simulink model "DC_Motor_model_closed_loop"  (R2026a)
settings: Solver=VariableStepAuto
model workspace (MAT data in the model file):
  B = Simulink.Parameter
  B.Value = 0.0001
  B.Complexity = 'real'
  B.Dimensions = [1 1]
  B.DataType = 'auto'
  J = Simulink.Parameter
  J.Value = 5e-05
  J.Complexity = 'real'
  J.Dimensions = [1 1]
  J.DataType = 'auto'
  Ke = Simulink.Parameter
  Ke.Value = 0.012
  Ke.Complexity = 'real'
  Ke.Dimensions = [1 1]
  Ke.DataType = 'auto'
  Kt = Simulink.Parameter
  Kt.Value = 0.012
  Kt.Complexity = 'real'
  Kt.Dimensions = [1 1]
  Kt.DataType = 'auto'
  L = Simulink.Parameter
  L.Value = 0.01
  L.Complexity = 'real'
  L.Dimensions = [1 1]
  L.DataType = 'auto'
  R = Simulink.Parameter
  R.Value = 5
  R.Complexity = 'real'
  R.Dimensions = [1 1]
  R.DataType = 'auto'
  TL = Simulink.Parameter
  TL.Value = 0
  TL.Complexity = 'real'
  TL.Dimensions = [1 1]
  TL.DataType = 'auto'
libraries: slpidlib x1

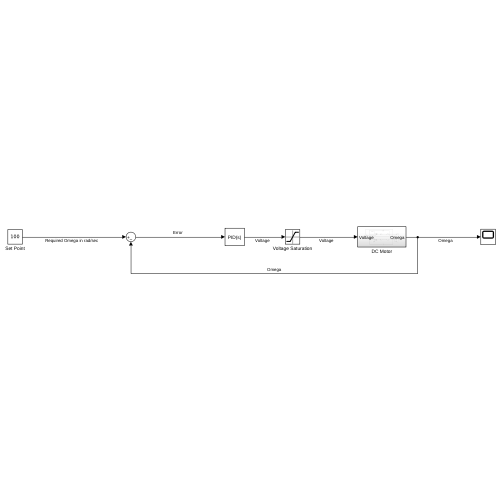
[thumbnail: Simulink's stored preview of the top-level diagram]
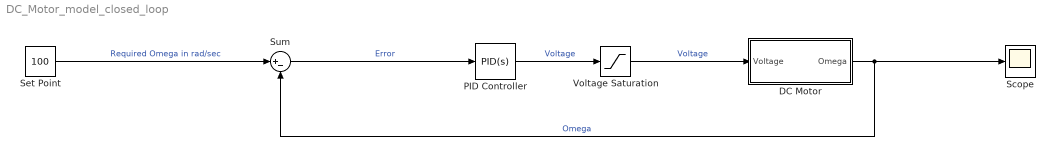
== system DC_Motor_model_closed_loop ==
  DC Motor : Subsystem
  PID Controller : slpidlib/PID Controller  Controller=PID  Form=Parallel  TimeDomain=Continuous-time  UseExternalTs=off  SampleTime=-1  IntegratorMethod=Forward Euler  FilterMethod=Forward Euler  ControllerParametersSource=internal  P=0.04  I=0.2  UseKiTs=off  D=0  UseExternalDerivativeSource=off  N=100  UseFilter=on  TunerSelectOption=Transfer Function Based (PID Tuner App)  InitialConditionSource=internal  InitialConditionForIntegrator=0  InitialConditionForFilter=0  DifferentiatorICPrevScaledInput=0  ExternalReset=none  TrackingMode=off  Kt=1  LimitOutput=off  SatLimitsSource=internal  UpperSaturationLimit=inf  LowerSaturationLimit=-inf  LinearizeAsGain=on  AntiWindupMode=none  Kb=1  LimitIntegrator=off  UpperIntegratorSaturationLimit=inf  LowerIntegratorSaturationLimit=-inf  POutMin=[]  POutMax=[]  IOutMin=[]  IOutMax=[]  DOutMin=[]  DOutMax=[]  NOutMin=[]  NOutMax=[]  SumOutMin=[]  SumOutMax=[]  SaturationOutMin=[]  SaturationOutMax=[]  PParamMin=[]  PParamMax=[]  IParamMin=[]  IParamMax=[]  DParamMin=[]  DParamMax=[]  NParamMin=[]  NParamMax=[]  KbParamMin=[]  KbParamMax=[]  KtParamMin=[]  KtParamMax=[]  KbOutMin=[]  KbOutMax=[]  KtOutMin=[]  KtOutMax=[]  IntegratorOutMin=[]  IntegratorOutMax=[]  FilterOutMin=[]  FilterOutMax=[]  SumI1OutMin=[]  SumI1OutMax=[]  SumI2OutMin=[]  SumI2OutMax=[]  SumI3OutMin=[]  SumI3OutMax=[]  SumI4OutMin=[]  SumI4OutMax=[]  SumDOutMin=[]  SumDOutMax=[]  DifferentiatorOutMin=[]  DifferentiatorOutMax=[]  FilterDiffOutCoefMin=[]  FilterDiffOutCoefMax=[]  ReciprocalOutMin=[]  ReciprocalOutMax=[]  SumDenOutMin=[]  SumDenOutMax=[]  SumNumOutMin=[]  SumNumOutMax=[]  DivideOutMin=[]  DivideOutMax=[]  UdiffTsProdOutMin=[]  UdiffTsProdOutMax=[]  NTsProdOutMin=[]  NTsProdOutMax=[]  UintegralTsProdOutMin=[]  UintegralTsProdOutMax=[]  UngainTsProdOutMin=[]  UngainTsProdOutMax=[]  ClampingZeroOutDataTypeStr=Inherit: Inherit via back propagation  ClampingZeroOutMin=[]  ClampingZeroOutMax=[]  FilterDenConstantOutDataTypeStr=Inherit: Inherit via back propagation  FilterDenConstantOutMin=[]  FilterDenConstantOutMax=[]  PCopyOutDataTypeStr=Inherit: Inherit via back propagation  PCopyOutMin=[]  PCopyOutMax=[]  NCopyOutDataTypeStr=Inherit: Inherit via back propagation  NCopyOutMin=[]  NCopyOutMax=[]  IntegratorContinuousStateAttributes=''  IntegratorStateMustResolveToSignalObject=off  IntegratorRTWStateStorageClass=Auto  FilterContinuousStateAttributes=''  FilterStateMustResolveToSignalObject=off  FilterRTWStateStorageClass=Auto  ParallelPVariant=InternalParameters  IdealPVariant=Disabled  IVariant=InternalParameters  DVariant=InternalParameters  IntegratorVariant=Continuous  SatVariant=Disabled  AWVariant=Passthrough  PCopyVariant=Disabled  TRVariant=Disabled  FdbkBlocksVariant=Forward  IdealPFdbkVariant=Disabled  SatFdbkVariant=Disabled  DerivativeFilterVariant=ContFilter  NVariant=InternalParameters  NCopyVariant=Disabled  FilterICVariant=InternalICsFilter  IntegratorICVariant=InternalICs  ExternalResetVariant=Disabled  TRSumVariant=Passthrough  SumFdbkVariant=Disabled  SumVariant=Sum_PID  TsampFilterVariant=InternalTs  TsampNgainVariant=Passthrough  TsampIntegralVariant=Disabled_SignalSpec  ExternalSaturationOutDataTypeStr=Inherit: Same as second input  DerivativeSourceVariant=ErrorSignal  PreIntVariant=InternalPreInt
  Scope : Scope
      settings: ActiveDisplayYMinimum=-13.144303855447449  ActiveDisplayYMaximum=118.29873469902707  DataLoggingVariableName=ScopeData2
  Set Point : Constant  Value=100
  Sum : Sum  Inputs=|+-
  Voltage Saturation : Saturate  UpperLimit=12  LowerLimit=0
  wires:
  Sum/1 -> PID Controller/1  "Error"
  Set Point/1 -> Sum/1  "Required Omega in rad/sec"
  DC Motor/1(Omega) -> Scope/1, Sum/2  "Omega"
  PID Controller/1 -> Voltage Saturation/1  "Voltage"
  Voltage Saturation/1 -> DC Motor/1(Voltage)  "Voltage"

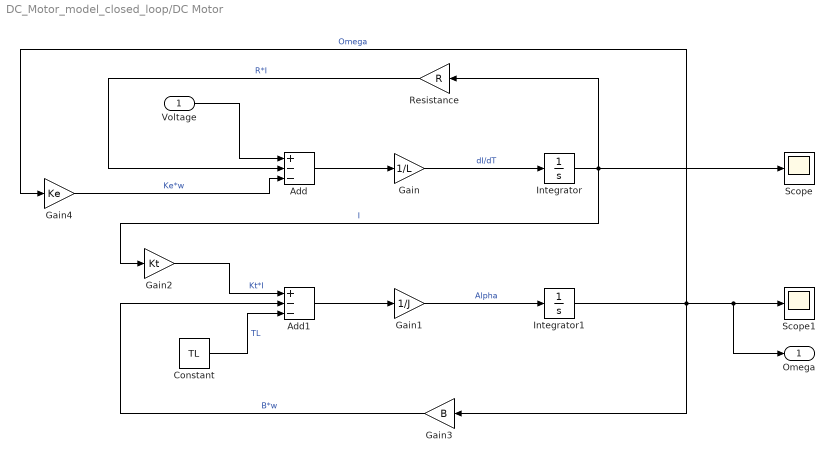
== system DC_Motor_model_closed_loop/DC Motor ==
  Voltage : Inport
  Add : Sum  Inputs=+--
  Add1 : Sum  Inputs=+--
  Constant : Constant  Value=TL
  Gain : Gain  Gain=1/L
  Gain1 : Gain  Gain=1/J
  Gain2 : Gain  Gain=Kt
  Gain3 : Gain  Gain=B
  Gain4 : Gain  Gain=Ke
  Integrator : Integrator
  Integrator1 : Integrator
  Resistance : Gain  Gain=R
  Scope : Scope
      settings: ActiveDisplayYMinimum=-0.29789795118869822  ActiveDisplayYMaximum=2.6810815606982845
  Scope1 : Scope
      settings: ActiveDisplayYMinimum=-27.950460827084147  ActiveDisplayYMaximum=251.55414744375739
  Omega : Outport
  wires:
  Resistance/1 -> Add/2  "R*I"
  Gain1/1 -> Integrator1/1  "Alpha"
  Add1/1 -> Gain1/1
  Integrator/1 -> Resistance/1, Scope/1, Gain2/1  "I"
  Integrator1/1 -> Omega/1, Scope1/1, Gain4/1, Gain3/1  "Omega"
  Gain4/1 -> Add/3  "Ke*w"
  Add/1 -> Gain/1
  Gain3/1 -> Add1/2  "B*w"
  Constant/1 -> Add1/3  "TL"
  Gain/1 -> Integrator/1  "dI/dT"
  Voltage/1 -> Add/1
  Gain2/1 -> Add1/1  "Kt*I"
